simulink subsystem "BatteryHV_Foundation_refsub"  (R2026a)
settings: Solver=VariableStepAuto
libraries: fl_lib x3
settings Model: Creator=isaacito  LastModifiedBy=isaacito

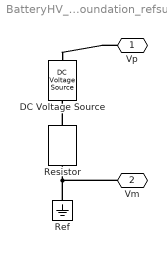
== system BatteryHV_Foundation_refsub ==
  DC Voltage Source : fl_lib/Electrical/Electrical Sources/DC Voltage Source  v0=400 V
  Ref : fl_lib/Electrical/Electrical Elements/Electrical Reference
  Resistor : fl_lib/Electrical/Electrical Elements/Resistor  R=0.01 Ohm  i_specify=off  i_priority=None  i=0 A  i_nominal_specify=off  i_nominal_value=1  i_nominal_unit=A  v_specify=off  v_priority=None  v=0 V  v_nominal_specify=off  v_nominal_value=1  v_nominal_unit=V
  Vp : PMIOPort  Side=Left
  Vm : PMIOPort  Port=2  Side=Left
  connections:
  Resistor/LConn1 -- DC Voltage Source/RConn1
  Ref/LConn1 -- Vm/RConn1 -- Resistor/RConn1
  Vp/RConn1 -- DC Voltage Source/LConn1
